simulink model "e3_1"  (R2022a)
settings: Solver=VariableStepAuto  StartTime=0.0  StopTime=10.0  RelTol=1e-3
settings Model: Creator=18075  LastModifiedBy=18075

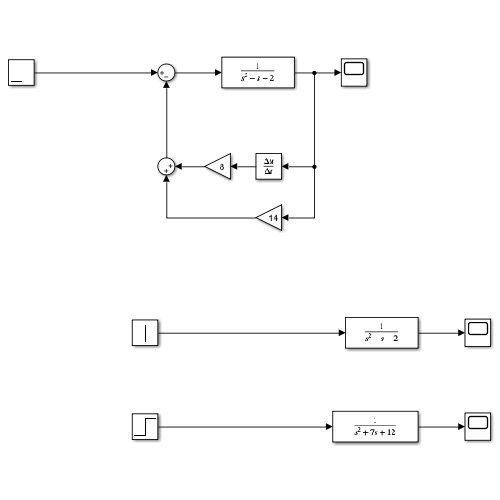
[thumbnail: Simulink's stored preview of the top-level diagram]
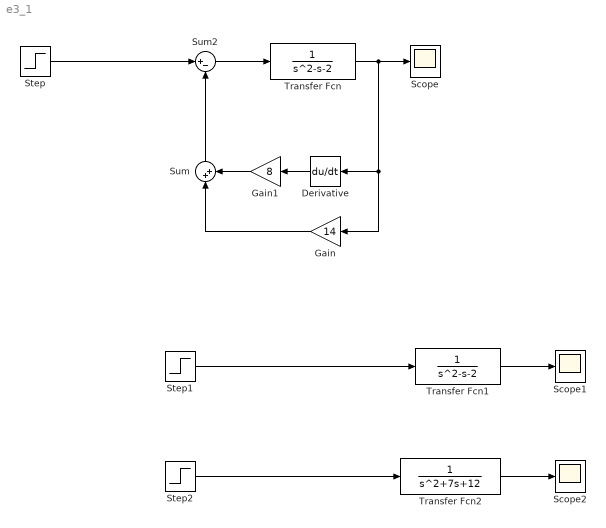
== system e3_1 ==
  Derivative : Derivative
  Gain : Gain  Gain=14
  Gain1 : Gain  Gain=8
  Scope : Scope
  Scope1 : Scope
  Scope2 : Scope
  Step : Step  SampleTime=0
  Step1 : Step  SampleTime=0
  Step2 : Step  SampleTime=0
  Sum : Sum  Inputs=|++
  Sum2 : Sum  Inputs=|+-
  Transfer Fcn : TransferFcn  Denominator=[1 -1 -2]
  Transfer Fcn1 : TransferFcn  Denominator=[1 -1 -2]
  Transfer Fcn2 : TransferFcn  Denominator=[1 7 12]
  wires:
  Step/1 -> Sum2/1
  Sum2/1 -> Transfer Fcn/1
  Transfer Fcn/1 -> Gain/1, Derivative/1, Scope/1
  Derivative/1 -> Gain1/1
  Sum/1 -> Sum2/2
  Gain/1 -> Sum/1
  Gain1/1 -> Sum/2
  Transfer Fcn1/1 -> Scope1/1
  Step1/1 -> Transfer Fcn1/1
  Transfer Fcn2/1 -> Scope2/1
  Step2/1 -> Transfer Fcn2/1
